simulink model "adrc_c_model"  (R2019b)
settings: Solver=FixedStepDiscrete  StartTime=0.0  StopTime=10.0  FixedStep=Ts  RelTol=1e-3
PreLoadFcn:
  | Ts = 0.001
InitFcn:
  | Ts = 0.001
  | mex controller.c
undefined symbols (not defined in the file): DiscIntNeverNeededParam
libraries: adrc x1, motion x1
settings Model: Creator=Kamran  LastModifiedBy=Kamran

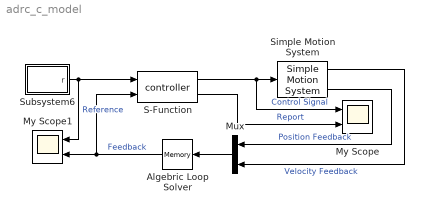
== system adrc_c_model ==
  Algebric Loop Solver : Memory
  Mux : Mux  Inputs=2
  My Scope : Scope  NumInputPorts=2
  My Scope1 : Scope  NumInputPorts=2
  S-Function : S-Function  FunctionName=controller  Parameters=Ts  SFunctionDeploymentMode=off  EnableBusSupport=off
  Simple Motion System : adrc/Simple Motion System  I=2  K=0.2  Taw=1e-3  Ts=Ts
  Subsystem6 : Subsystem
      mask Display: disp("Profile")
  wires:
  S-Function/1 -> My Scope/1, Simple Motion System/1  "Control Signal"
  S-Function/2 -> My Scope/2  "Report"
  Simple Motion System/2 -> Mux/1  "Position Feedback"
  Simple Motion System/1 -> Mux/2  "Velocity Feedback"
  Mux/1 -> Algebric Loop Solver/1
  Subsystem6/1(r) -> S-Function/1, My Scope1/1  "Reference"
  Algebric Loop Solver/1 -> My Scope1/2, S-Function/2  "Feedback"

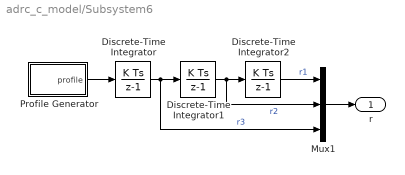
== system adrc_c_model/Subsystem6 ==
  Discrete-Time Integrator : DiscreteIntegrator  SampleTime=-1  ICPrevOutput=DiscIntNeverNeededParam  ICPrevScaledInput=DiscIntNeverNeededParam
  Discrete-Time Integrator1 : DiscreteIntegrator  SampleTime=-1  ICPrevOutput=DiscIntNeverNeededParam  ICPrevScaledInput=DiscIntNeverNeededParam
  Discrete-Time Integrator2 : DiscreteIntegrator  SampleTime=-1  ICPrevOutput=DiscIntNeverNeededParam  ICPrevScaledInput=DiscIntNeverNeededParam
  Mux1 : Mux  Inputs=3
  Profile Generator : Subsystem  BlockChoice=Jerk
      link override Jerk: t0=1  x=2  a=2  j=3  Ts=Ts
      settings: AttributesFormatString=%<BlockChoice>  TemplateBlock=motion/Profile Generators/Profile Generator  MemberBlocks=Acceleration,Derivative of Jerk,Jerk,dJerk with error correction
  r : Outport
  wires:
  Profile Generator/1(profile) -> Discrete-Time Integrator/1
  Discrete-Time Integrator1/1 -> Mux1/2, Discrete-Time Integrator2/1  "r2"
  Discrete-Time Integrator/1 -> Mux1/3, Discrete-Time Integrator1/1  "r3"
  Mux1/1 -> r/1
  Discrete-Time Integrator2/1 -> Mux1/1  "r1"

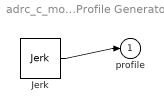
== system adrc_c_model/Subsystem6/Profile Generator ==
  Jerk : motion/Profile Generators/Jerk  t0=1  x=2  v=1  a=2  j=3  Ts=Ts
  profile : Outport
  wires:
  Jerk/1 -> profile/1
